simulink model "linear2_model"  (R2012b)
settings: Solver=ode45  StartTime=0.0  StopTime=10.0  RelTol=1e-3
settings Model: BufferReuse=off  Creator=stsuei  LastModifiedBy=stsuei
settings DataIOCC: ExternalInput=[0 0.87449459647241 0]  InitialState=[]  LoadExternalInput=on  LoadInitialState=on
settings OptimizationCC: InlineParams=on  BufferReuse=off
settings DebuggingCC: SolverPrmCheckMsg=none  InitInArrayFormatMsg=none

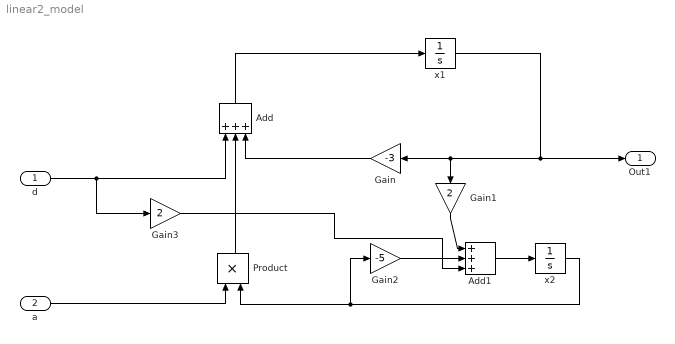
== system linear2_model ==
  d : Inport
  a : Inport  Port=2
  Add : Sum  Inputs=+++
  Add1 : Sum  Inputs=+++
  Gain : Gain  Gain=-3
  Gain1 : Gain  Gain=2
  Gain2 : Gain  Gain=-5
  Gain3 : Gain  Gain=2
  Product : Product  RndMeth=Zero
  x1 : Integrator
  x2 : Integrator
  Out1 : Outport
  wires:
  x1/1 -> Gain1/1, Gain/1, Out1/1
  x2/1 -> Gain2/1, Product/2
  a/1 -> Product/1
  Add/1 -> x1/1
  Product/1 -> Add/2
  Gain/1 -> Add/3
  d/1 -> Gain3/1, Add/1
  Add1/1 -> x2/1
  Gain2/1 -> Add1/3
  Gain3/1 -> Add1/2
  Gain1/1 -> Add1/1
